simulink model "test"  (R2020b)
settings: Solver=ode4  StartTime=0.0  StopTime=inf  FixedStep=1/1000  RelTol=1e-3
libraries: speedgoatlib_IO691 x8, canmsglib x6, simulink x2
(part 1 of 2)
settings Model: SimulationMode=external  ExtModeEnableFloating=off  Creator=Mechatronics  LastModifiedBy=Mechatronics
settings SolverCC: ConcurrentTasks=on  PositivePriorityOrder=on
settings OptimizationCC: BlockReduction=off  OptimizeBlockIOStorage=off
settings DebuggingCC: TasksWithSamePriorityMsg=none
settings HardwareCC: ProdBitPerLong=64  ProdLongLongMode=on  ProdHWDeviceType=Intel->x86-64 (Linux 64)
settings RTWCC: Description=Simulink Real-Time  SystemTargetFile=slrealtime.tlc  TemplateMakefile=slrealtime_default_tmf  Toolchain=Simulink Real-Time Toolchain  BuildConfiguration=Faster Runs  CodeExecutionProfiling=on  TargetLang=C++

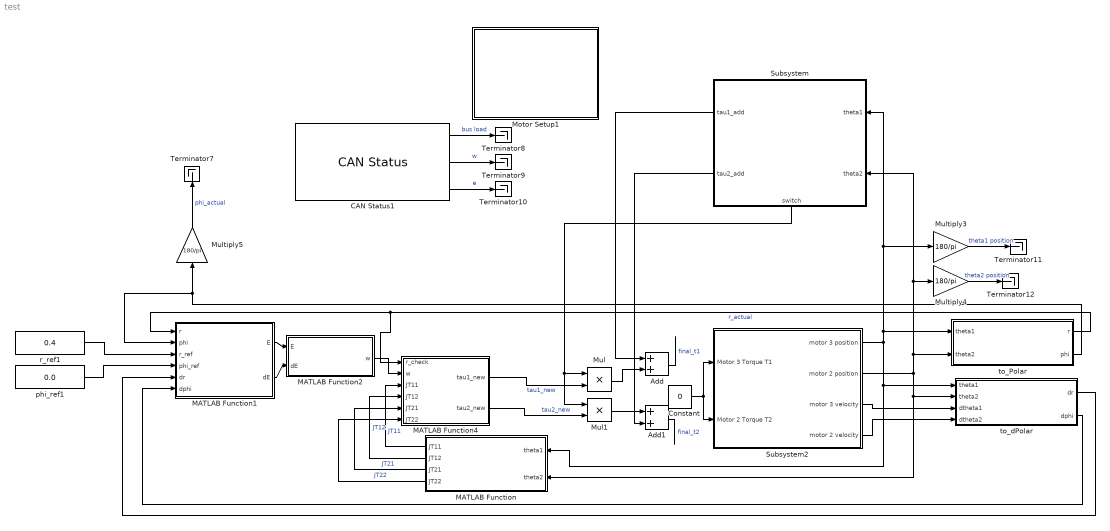
== system test ==
  Add : Sum
  Add1 : Sum
  CAN Status1 : speedgoatlib_IO691/CAN Status  moduleId=1  sampleTime=-1  channel=1  busRecovery=Off  arrayOutput=off  controllerCpuLoad=off  controllerLiveCount=off  initModeAct=off  avgBusLoad=on  receiving=off  RxQueueEmpty=off  dataOverrunRcv=off  rxBufferLevel=off  txPending=off  dataOverrunTx=off  txBufferLevel=off  errWarnLimit=on  errPassLimit=on  errBusOff=off  busRecoveryCounter=off  busCouplingErr=off  transceiverErr=off  opMode=off  brp=off  timeSegment1=off  timeSegment2=off  synchronisationJumpWidth=off  dataTSEG1=off  dataTSEG2=off  dataSJW=off  moduleType=691  qtyStatBlk=1  ptIdx=0  isFDMod=0
      settings: SourceProductName=Simulink Real-Time: Speedgoat I/O Blockset
  Constant : Constant  Value=0
  MATLAB Function : MATLAB Function  TreatAsAtomicUnit=on
  MATLAB Function1 : MATLAB Function  TreatAsAtomicUnit=on
  MATLAB Function2 : MATLAB Function  TreatAsAtomicUnit=on
  MATLAB Function4 : MATLAB Function  TreatAsAtomicUnit=on
  Motor Setup1 : Subsystem
  Mul : Product  Inputs=**
  Mul1 : Product  Inputs=**
  Multiply3 : Gain  Gain=180/pi
  Multiply4 : Gain  Gain=180/pi
  Multiply5 : Gain  Gain=180/pi
  Subsystem : Subsystem
      settings: PortSchema="{\"entries\":[{\"content\":{\"sides\":[{\"content\":{\"connectorIds\":[\"In1\",\"In2\"]},\"type\":\"ConnectorPlacement.EquallySpacedRectSide\",\"uuid\":\"133de2dd-f27a-4cc1-bddd-d1f84e4836c9\"},{\"content\":{\"connectorIds\":[\"Out1\",\"Out2\"],\"side\":\"RIGHT\"},\"type\":\"ConnectorPlacement.EquallySpacedRectSide\",\"uuid\":\"6569a8f1-8858-49fe-b592-3edc35f7d01c\"},{\"content\":{\"connectorIds\":[],\"side\":\"TOP\"},\"type\":\"ConnectorPlacement.EquallySpacedRectSide\",\"uuid\":\"dbb559e8-791c-4587-9e9a-4749d8cc79c6\"},{\"content\":{\"connectorIds\":[\"Out3\"],\"side\":\"BOTTOM\"},\"type\":\"ConnectorPlacement.EquallySpacedRectSide\",\"uuid\":\"b7c4d305-876d-4161-8903-ada4b7512b16\"},{\"content\":{\"connectorIds\":[],\"side\":\"HIDDEN\"},\"type\":\"ConnectorPlacement.EquallySpacedRectSide\",\"uuid\":\"a0aadd7d-61d3-4ce9-a370-27d87e201b6f\"}]},\"type\":\"ConnectorPlacement.EquallySpacedConnector\",\"uuid\":\"543a852a-1c67-4df2-af33-899992a7334e\"}],\"packageUris\":[\"http://schema.mathworks.com/mf0/Connector/R2020b\"],\"version\":\"1.0\"}"
  Subsystem2 : Subsystem
  Terminator{7..12} (6 alike) : Terminator
  phi_ref1 : Constant  Value=0.0
  r_ref1 : Constant  Value=0.4
  to_Polar : MATLAB Function  TreatAsAtomicUnit=on
  to_dPolar : MATLAB Function  TreatAsAtomicUnit=on
  wires:
  MATLAB Function4/2(tau2_new) -> Mul1/2  "tau2_new"
  Add/1 -> ?  "final_t1"
  Subsystem/3(switch) -> Mul1/1, Mul/1
  Multiply5/1 -> Terminator7/1  "phi_actual"
  Subsystem2/2(motor 2 position) -> to_dPolar/2(theta2), MATLAB Function/2(theta2), to_Polar/2(theta2), Subsystem/2(theta2), Multiply4/1
  MATLAB Function4/1(tau1_new) -> Mul/2  "tau1_new"
  Mul1/1 -> Add1/1
  MATLAB Function/4(JT22) -> MATLAB Function4/6(JT22)  "JT22"
  MATLAB Function/3(JT21) -> MATLAB Function4/5(JT21)  "JT21"
  MATLAB Function2/1(w) -> MATLAB Function4/2(w)
  Multiply4/1 -> Terminator12/1  "theta2 position"
  Multiply3/1 -> Terminator11/1  "theta1 position"
  MATLAB Function/2(JT12) -> MATLAB Function4/4(JT12)  "JT12"
  Subsystem/1(tau1_add) -> Add/1
  Subsystem2/3(motor 3 velocity) -> to_dPolar/3(dtheta1)
  Subsystem2/4(motor 2 velocity) -> to_dPolar/4(dtheta2)
  MATLAB Function/1(JT11) -> MATLAB Function4/3(JT11)  "JT11"
  Subsystem/2(tau2_add) -> Add1/2
  to_dPolar/1(dr) -> MATLAB Function1/5(dr)
  to_Polar/2(phi) -> MATLAB Function1/2(phi), Multiply5/1
  CAN Status1/1 -> Terminator8/1  "bus load"
  to_dPolar/2(dphi) -> MATLAB Function1/6(dphi)
  Subsystem2/1(motor 3 position) -> to_dPolar/1(theta1), MATLAB Function/1(theta1), to_Polar/1(theta1), Subsystem/1(theta1), Multiply3/1
  r_ref1/1 -> MATLAB Function1/3(r_ref)
  CAN Status1/3 -> Terminator10/1  "e"
  Add1/1 -> ?  "final_t2"
  MATLAB Function1/2(dE) -> MATLAB Function2/2(dE)
  MATLAB Function1/1(E) -> MATLAB Function2/1(E)
  to_Polar/1(r) -> MATLAB Function4/1(r_check), MATLAB Function1/1(r)  "r_actual"
  Mul/1 -> Add/2
  CAN Status1/2 -> Terminator9/1  "w"
  phi_ref1/1 -> MATLAB Function1/4(phi_ref)
  Constant/1 -> Subsystem2/2(Motor 2 Torque T2), Subsystem2/1(Motor 3 Torque T1)

== system test/Motor Setup1 ==
  CAN setup : speedgoatlib_IO691/CAN Setup   moduletype=IO691  id=1  pciSlot=-1  chn1=CAN (HS)  chn2=Disabled  chn3=Disabled  chn4=Disabled  initStruct=[]  termStruct=[struct('Channel',1,'Protocol','CAN','BRS',0,'Type','Standard','Identifier',2,'Data',[255, 255, 255, 255, 255, 255, 255, 253],'Pause',0.001), struct('Channel',1,'Protocol','CAN','BRS',0,'Type','Standard','Identifier',3,'Data',[255, 255, 255, 255, 255, 255, 255, 253],'Pause',0.001)]  ArbitrationbdrChn1=1.0 MBaud  ArbitrationManbdrChn1=[2,8,31,8]  FdbdrChn1=1.0 MBaud  FdManbdrChn1=[2,8,31,8]  ArbitrationbdrChn2=1.0 MBaud  ArbitrationManbdrChn2=[2,8,31,8]  FdbdrChn2=1.0 MBaud  FdManbdrChn2=[2,8,31,8]  ArbitrationbdrChn3=1.0 MBaud  ArbitrationManbdrChn3=[2,8,31,8]  FdbdrChn3=5.0 MBaud  FdManbdrChn3=[2,2,5,2]  ArbitrationbdrChn4=1.0 MBaud  ArbitrationManbdrChn4=[2,8,31,8]  FdbdrChn4=5.0 MBaud  FdManbdrChn4=[2,2,5,2]  moduleInitValues=[691 1 -1 -1]
      settings: SourceProductName=Simulink Real-Time: Speedgoat I/O Blockset
  Motor Setup : Subsystem

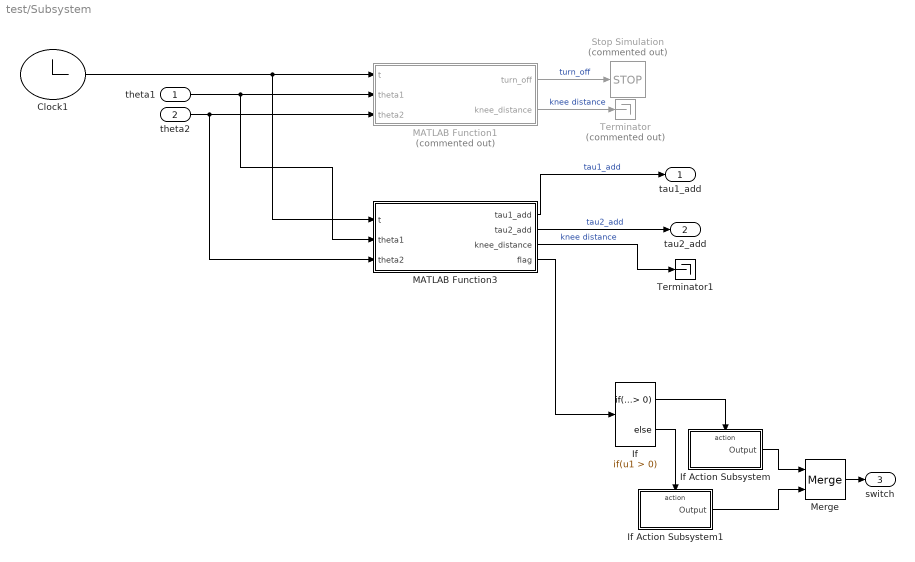
== system test/Subsystem ==
  theta1 : Inport
  theta2 : Inport  Port=2
  Clock1 : Clock
  If : If
  If Action Subsystem : Subsystem  TreatAsAtomicUnit=on
  If Action Subsystem1 : Subsystem  TreatAsAtomicUnit=on
  MATLAB Function1 : MATLAB Function  Commented=on  TreatAsAtomicUnit=on
  MATLAB Function3 : MATLAB Function  TreatAsAtomicUnit=on
  Merge : Merge
  Stop Simulation : Stop  Commented=on
  Terminator : Terminator  Commented=on
  Terminator1 : Terminator
  tau1_add : Outport
  tau2_add : Outport  Port=2
  switch : Outport  Port=3
  wires:
  theta2/1 -> MATLAB Function3/3(theta2), MATLAB Function1/3(theta2)
  theta1/1 -> MATLAB Function3/2(theta1), MATLAB Function1/2(theta1)
  MATLAB Function3/2(tau2_add) -> tau2_add/1  "tau2_add"
  MATLAB Function3/1(tau1_add) -> tau1_add/1  "tau1_add"
  MATLAB Function1/2(knee_distance) -> Terminator/1  "knee distance"
  MATLAB Function1/1(turn_off) -> Stop Simulation/1  "turn_off"
  Clock1/1 -> MATLAB Function3/1(t), MATLAB Function1/1(t)
  MATLAB Function3/3(knee_distance) -> Terminator1/1  "knee distance"
  If/2 -> If Action Subsystem1/Action
  If/1 -> If Action Subsystem/Action
  MATLAB Function3/4(flag) -> If/1
  If Action Subsystem/1(Output) -> Merge/1
  If Action Subsystem1/1(Output) -> Merge/2
  Merge/1 -> switch/1

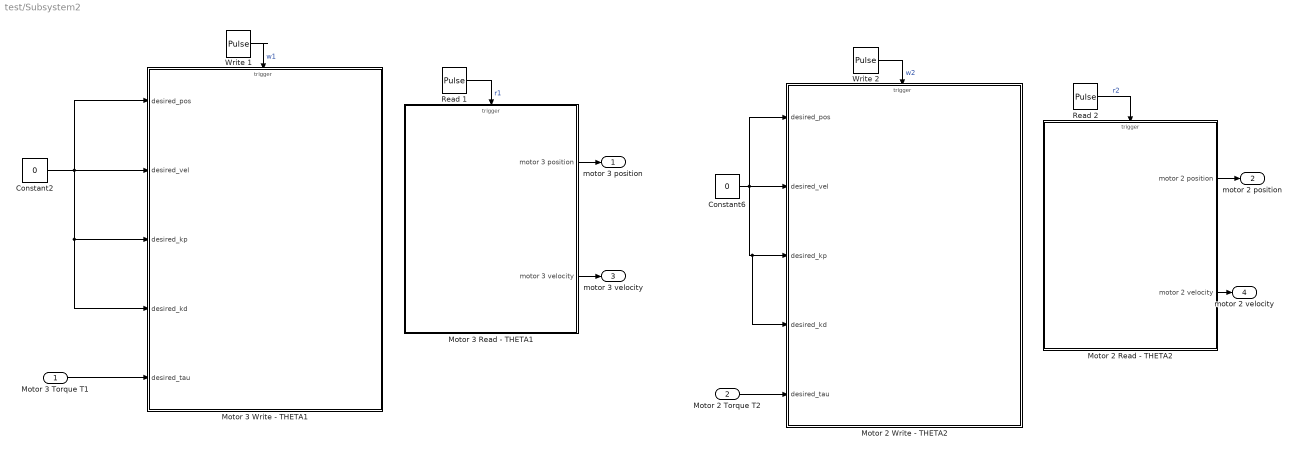
== system test/Subsystem2 ==
  Motor 3 Torque T1 : Inport
  Motor 2 Torque T2 : Inport  Port=2
  Constant2 : Constant  Value=0
  Constant6 : Constant  Value=0
  Motor 2 Read - THETA2 : Subsystem
  Motor 2 Write - THETA2 : Subsystem  TreatAsAtomicUnit=on
  Motor 3 Read - THETA1 : Subsystem
  Motor 3 Write - THETA1 : Subsystem  TreatAsAtomicUnit=on
  Read 1 : DiscretePulseGenerator  PulseType=Time based  Period=1/250  PulseWidth=50  PhaseDelay=3.001
  Read 2 : DiscretePulseGenerator  PulseType=Time based  Period=1/250  PulseWidth=50  PhaseDelay=3.003
  Write 1 : DiscretePulseGenerator  PulseType=Time based  Period=1/250  PulseWidth=50  PhaseDelay=3
  Write 2 : DiscretePulseGenerator  PulseType=Time based  Period=1/250  PulseWidth=50  PhaseDelay=3.002
  motor 3 position : Outport
  motor 2 position : Outport  Port=2
  motor 3 velocity : Outport  Port=3
  motor 2 velocity : Outport  Port=4
  wires:
  Motor 3 Read - THETA1/1(motor 3 position) -> motor 3 position/1
  Write 2/1 -> Motor 2 Write - THETA2/Trigger  "w2"
  Motor 2 Torque T2/1 -> Motor 2 Write - THETA2/5(desired_tau)
  Motor 2 Read - THETA2/2(motor 2 velocity) -> motor 2 velocity/1
  Motor 3 Read - THETA1/2(motor 3 velocity) -> motor 3 velocity/1
  Read 2/1 -> Motor 2 Read - THETA2/Trigger  "r2"
  Motor 3 Torque T1/1 -> Motor 3 Write - THETA1/5(desired_tau)
  Motor 2 Read - THETA2/1(motor 2 position) -> motor 2 position/1
  Read 1/1 -> Motor 3 Read - THETA1/Trigger  "r1"
  Write 1/1 -> Motor 3 Write - THETA1/Trigger  "w1"
  Constant6/1 -> Motor 2 Write - THETA2/1(desired_pos), Motor 2 Write - THETA2/4(desired_kd), Motor 2 Write - THETA2/3(desired_kp), Motor 2 Write - THETA2/2(desired_vel)
  Constant2/1 -> Motor 3 Write - THETA1/1(desired_pos), Motor 3 Write - THETA1/2(desired_vel), Motor 3 Write - THETA1/4(desired_kd), Motor 3 Write - THETA1/3(desired_kp)

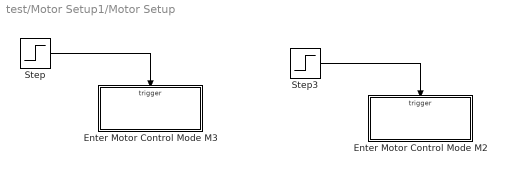
== system test/Motor Setup1/Motor Setup ==
  Enter Motor Control Mode M2 : Subsystem  TreatAsAtomicUnit=on
  Enter Motor Control Mode M3 : Subsystem  TreatAsAtomicUnit=on
  Step : Step  Time=1.0
  Step3 : Step  Time=2
  wires:
  Step3/1 -> Enter Motor Control Mode M2/Trigger
  Step/1 -> Enter Motor Control Mode M3/Trigger

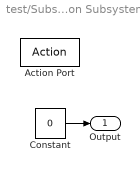
== system test/Subsystem/If Action Subsystem ==
  Action Port : ActionPort  ActionPortLabel=if(u1 > 0)
  Constant : Constant  Value=0
  Output : Outport
  wires:
  Constant/1 -> Output/1

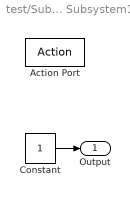
== system test/Subsystem/If Action Subsystem1 ==
  Action Port : ActionPort  ActionPortLabel=else
  Constant : Constant
  Output : Outport
  wires:
  Constant/1 -> Output/1

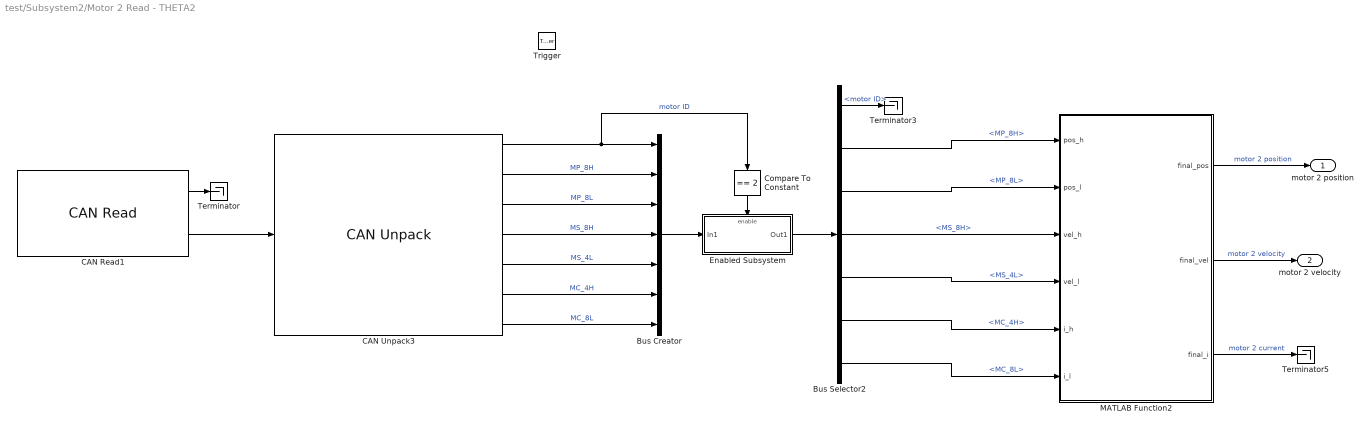
== system test/Subsystem2/Motor 2 Read - THETA2 ==
  Trigger : TriggerPort  VariantControl=Variant  PortDimensions=1
  Bus Creator : BusCreator  Inputs=7
  Bus Selector2 : BusSelector  OutputSignals=motor ID,MP_8H,MP_8L,MS_8H,MS_4L,MC_4H,MC_8L
  CAN Read1 : speedgoatlib_IO691/CAN Read  id=1  ts=-1  channel=1  messageType=CAN  canType=CAN (HS)  initValues=[691 1 -1 0 1 1]
      settings: SourceProductName=Simulink Real-Time: Speedgoat Library
  CAN Unpack3 : canmsglib/CAN Unpack  MsgList=(none)  MsgName=CAN Msg  MsgIDType=Standard (11-bit identifier)  MsgIdentifier=0  MsgLength=8  SignalInfo={ 'Drive ID', '0', '8', 'LE', 'unsigned', 'Standard', '0', '1', '0', '-Inf', 'Inf'; 'Motor position 8-H', '8', '8', 'LE', 'unsigned', 'Standard', '0', '1', '0', '-Inf', 'Inf'; 'Motor position 8-L', '16', '8', 'LE', 'unsigned', 'Standard', '0', '1', '0', '-Inf', 'Inf'; 'Motor speed 8-H', '24', '8', 'LE', 'unsigned', 'Standard', '0', '1', '0', '-Inf', 'Inf'; 'Motor speed 4-L', '36', '4', 'LE', 'unsigned', 'Standard', '0', '1', '0', '-Inf', 'Inf'; 'Current 4-H', '32', '4', 'LE', 'unsigned', 'Standard', '0', '1', '0', '-Inf', 'Inf'; 'Current 8-L', '40', '8', 'LE', 'unsigned', 'Standard', '0', '1', '0', '-Inf', 'Inf' }  IDPort=off  TimestampPort=off  ErrorPort=off  RemotePort=off  LengthPort=off  StatusPort=off  ApplyMinMax=off
      settings: SourceProductBaseCode=ME,XP,VN
  Compare To Constant : simulink/Logic and Bit Operations/Compare To Constant  relop===  const=2  OutDataTypeStr=boolean
  Enabled Subsystem : Subsystem  TreatAsAtomicUnit=on
  MATLAB Function2 : MATLAB Function  TreatAsAtomicUnit=on
  Terminator : Terminator
  Terminator3 : Terminator
  Terminator5 : Terminator
  motor 2 position : Outport
  motor 2 velocity : Outport  Port=2
  wires:
  MATLAB Function2/3(final_i) -> Terminator5/1  "motor 2 current"
  MATLAB Function2/1(final_pos) -> motor 2 position/1  "motor 2 position"
  MATLAB Function2/2(final_vel) -> motor 2 velocity/1  "motor 2 velocity"
  CAN Unpack3/7 -> Bus Creator/7  "MC_8L"
  Bus Selector2/4 -> MATLAB Function2/3(vel_h)  "<MS_8H>"
  Bus Selector2/7 -> MATLAB Function2/6(i_l)  "<MC_8L>"
  CAN Unpack3/4 -> Bus Creator/4  "MS_8H"
  CAN Unpack3/6 -> Bus Creator/6  "MC_4H"
  Bus Selector2/1 -> Terminator3/1  "<motor ID>"
  CAN Unpack3/3 -> Bus Creator/3  "MP_8L"
  Bus Selector2/2 -> MATLAB Function2/1(pos_h)  "<MP_8H>"
  Bus Selector2/5 -> MATLAB Function2/4(vel_l)  "<MS_4L>"
  CAN Unpack3/2 -> Bus Creator/2  "MP_8H"
  CAN Read1/2 -> CAN Unpack3/1
  CAN Unpack3/5 -> Bus Creator/5  "MS_4L"
  Bus Selector2/6 -> MATLAB Function2/5(i_h)  "<MC_4H>"
  Bus Selector2/3 -> MATLAB Function2/2(pos_l)  "<MP_8L>"
  Compare To Constant/1 -> Enabled Subsystem/Enable
  Bus Creator/1 -> Enabled Subsystem/1(In1)
  CAN Unpack3/1 -> Compare To Constant/1, Bus Creator/1  "motor ID"
  Enabled Subsystem/1(Out1) -> Bus Selector2/1
  CAN Read1/1 -> Terminator/1

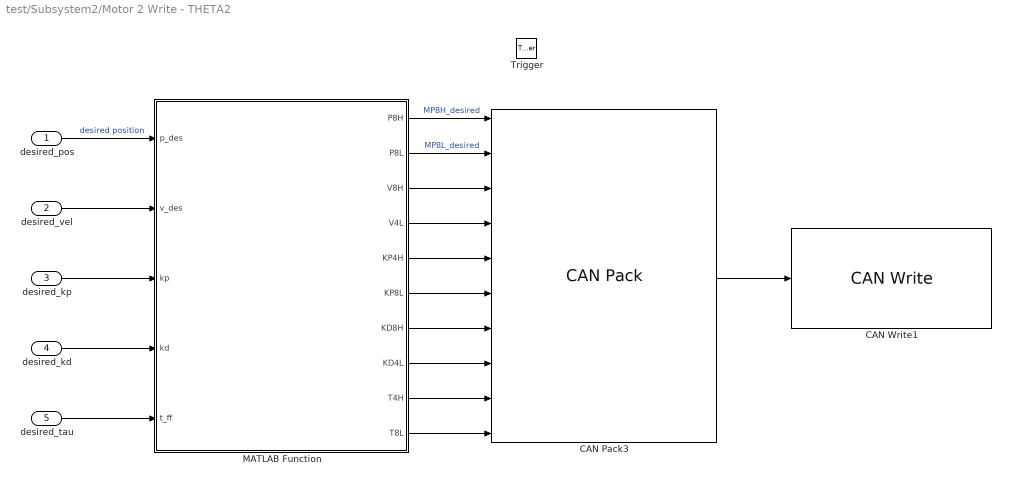
== system test/Subsystem2/Motor 2 Write - THETA2 ==
  desired_pos : Inport
  desired_vel : Inport  Port=2
  desired_kp : Inport  Port=3
  desired_kd : Inport  Port=4
  desired_tau : Inport  Port=5
  Trigger : TriggerPort  VariantControl=Variant
  CAN Pack3 : canmsglib/CAN Pack  MsgList=(none)  MsgName=MotorControl  MsgIDType=Standard (11-bit identifier)  MsgIdentifier=2  MsgLength=8  Remote=off  ApplyMinMax=off  BusOutput=off  SignalInfo={ 'Motor postition 8-H', '0', '8', 'LE', 'unsigned', 'Standard', '0', '1', '0', '-Inf', 'Inf'; 'Motor position 8-L', '8', '8', 'LE', 'unsigned', 'Standard', '0', '1', '0', '-Inf', 'Inf'; 'Motor speed 8-H', '16', '8', 'LE', 'unsigned', 'Standard', '0', '1', '0', '-Inf', 'Inf'; 'Motor speed 4-L', '28', '4', 'LE', 'unsigned', 'Standard', '0', '1', '0', '-Inf', 'Inf'; 'KP 4-H', '24', '4', 'LE', 'unsigned', 'Standard', '0', '1', '0', '-Inf', 'Inf'; 'KP 8-L', '32', '8', 'LE', 'unsigned', 'Standard', '0', '1', '0', '-Inf', 'Inf'; 'KD 8-H', '40', '8', 'LE', 'unsigned', 'Standard', '0', '1', '0', '-Inf', 'Inf'; 'KD 4-L', '52', '4', 'LE', 'unsigned', 'Standard', '0', '1', '0', '-Inf', 'Inf'; 'Current 4-H', '48', '4', 'LE', 'unsigned', 'Standard', '0', '1', '0', '-Inf', 'Inf'; 'Current 8-L', '56', '8', 'LE', 'unsigned', 'Standard', '0', '1', '0', '-Inf', 'Inf' }
      settings: SourceProductBaseCode=ME,XP,VN  DataFormat=manually specified signals
  CAN Write1 : speedgoatlib_IO691/CAN Write  id=1  ts=-1  channel=1  messageType=CAN  enableStatusPort=off  canType=CAN (HS)  initValues=[691 1 -1 0 1 1 0]
      settings: SourceProductName=Simulink Real-Time: Speedgoat Library
  MATLAB Function : MATLAB Function  TreatAsAtomicUnit=on
  wires:
  desired_vel/1 -> MATLAB Function/2(v_des)
  desired_pos/1 -> MATLAB Function/1(p_des)  "desired position"
  MATLAB Function/6(KP8L) -> CAN Pack3/6
  MATLAB Function/7(KD8H) -> CAN Pack3/7
  MATLAB Function/2(P8L) -> CAN Pack3/2  "MP8L_desired"
  desired_kp/1 -> MATLAB Function/3(kp)
  MATLAB Function/5(KP4H) -> CAN Pack3/5
  desired_kd/1 -> MATLAB Function/4(kd)
  desired_tau/1 -> MATLAB Function/5(t_ff)
  MATLAB Function/8(KD4L) -> CAN Pack3/8
  MATLAB Function/4(V4L) -> CAN Pack3/4
  MATLAB Function/9(T4H) -> CAN Pack3/9
  MATLAB Function/1(P8H) -> CAN Pack3/1  "MP8H_desired"
  CAN Pack3/1 -> CAN Write1/1
  MATLAB Function/3(V8H) -> CAN Pack3/3
  MATLAB Function/10(T8L) -> CAN Pack3/10

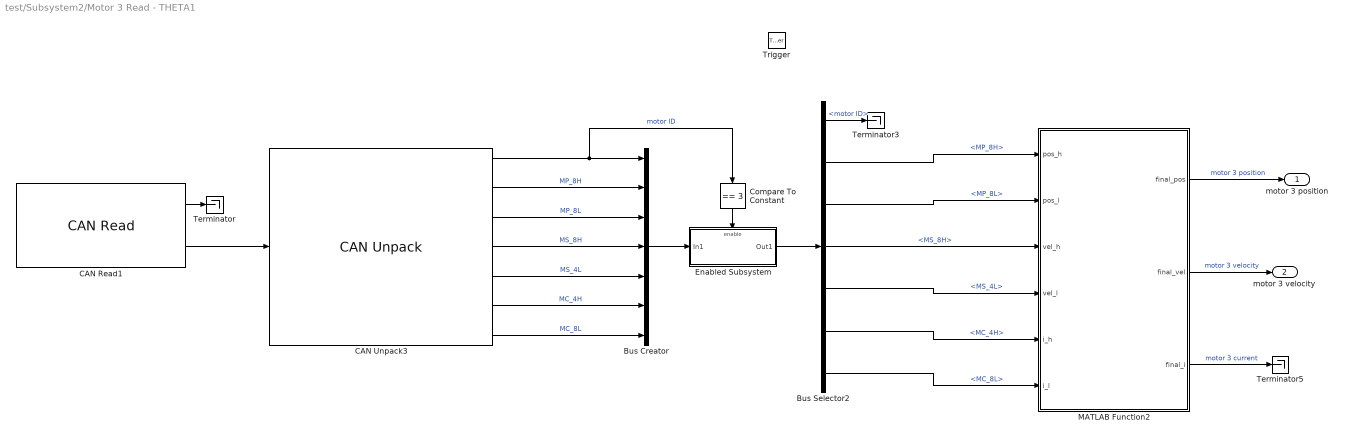
== system test/Subsystem2/Motor 3 Read - THETA1 ==
  Trigger : TriggerPort  VariantControl=Variant  PortDimensions=1
  Bus Creator : BusCreator  Inputs=7
  Bus Selector2 : BusSelector  OutputSignals=motor ID,MP_8H,MP_8L,MS_8H,MS_4L,MC_4H,MC_8L
  CAN Read1 : speedgoatlib_IO691/CAN Read  id=1  ts=-1  channel=1  messageType=CAN  canType=CAN (HS)  initValues=[691 1 -1 0 1 1]
      settings: SourceProductName=Simulink Real-Time: Speedgoat Library
  CAN Unpack3 : canmsglib/CAN Unpack  MsgList=(none)  MsgName=CAN Msg  MsgIDType=Standard (11-bit identifier)  MsgIdentifier=0  MsgLength=8  SignalInfo={ 'Drive ID', '0', '8', 'LE', 'unsigned', 'Standard', '0', '1', '0', '-Inf', 'Inf'; 'Motor position 8-H', '8', '8', 'LE', 'unsigned', 'Standard', '0', '1', '0', '-Inf', 'Inf'; 'Motor position 8-L', '16', '8', 'LE', 'unsigned', 'Standard', '0', '1', '0', '-Inf', 'Inf'; 'Motor speed 8-H', '24', '8', 'LE', 'unsigned', 'Standard', '0', '1', '0', '-Inf', 'Inf'; 'Motor speed 4-L', '36', '4', 'LE', 'unsigned', 'Standard', '0', '1', '0', '-Inf', 'Inf'; 'Current 4-H', '32', '4', 'LE', 'unsigned', 'Standard', '0', '1', '0', '-Inf', 'Inf'; 'Current 8-L', '40', '8', 'LE', 'unsigned', 'Standard', '0', '1', '0', '-Inf', 'Inf' }  IDPort=off  TimestampPort=off  ErrorPort=off  RemotePort=off  LengthPort=off  StatusPort=off  ApplyMinMax=off
      settings: SourceProductBaseCode=ME,XP,VN
  Compare To Constant : simulink/Logic and Bit Operations/Compare To Constant  relop===  const=3  OutDataTypeStr=boolean
  Enabled Subsystem : Subsystem  TreatAsAtomicUnit=on
  MATLAB Function2 : MATLAB Function  TreatAsAtomicUnit=on
  Terminator : Terminator
  Terminator3 : Terminator
  Terminator5 : Terminator
  motor 3 position : Outport
  motor 3 velocity : Outport  Port=2
  wires:
  MATLAB Function2/3(final_i) -> Terminator5/1  "motor 3 current"
  MATLAB Function2/1(final_pos) -> motor 3 position/1  "motor 3 position"
  MATLAB Function2/2(final_vel) -> motor 3 velocity/1  "motor 3 velocity"
  CAN Unpack3/7 -> Bus Creator/7  "MC_8L"
  Bus Selector2/4 -> MATLAB Function2/3(vel_h)  "<MS_8H>"
  Bus Selector2/7 -> MATLAB Function2/6(i_l)  "<MC_8L>"
  CAN Unpack3/4 -> Bus Creator/4  "MS_8H"
  CAN Unpack3/6 -> Bus Creator/6  "MC_4H"
  Bus Selector2/1 -> Terminator3/1  "<motor ID>"
  CAN Unpack3/3 -> Bus Creator/3  "MP_8L"
  Bus Selector2/2 -> MATLAB Function2/1(pos_h)  "<MP_8H>"
  Bus Selector2/5 -> MATLAB Function2/4(vel_l)  "<MS_4L>"
  CAN Unpack3/2 -> Bus Creator/2  "MP_8H"
  CAN Read1/2 -> CAN Unpack3/1
  CAN Unpack3/5 -> Bus Creator/5  "MS_4L"
  Bus Selector2/6 -> MATLAB Function2/5(i_h)  "<MC_4H>"
  Bus Selector2/3 -> MATLAB Function2/2(pos_l)  "<MP_8L>"
  Compare To Constant/1 -> Enabled Subsystem/Enable
  Bus Creator/1 -> Enabled Subsystem/1(In1)
  CAN Unpack3/1 -> Compare To Constant/1, Bus Creator/1  "motor ID"
  Enabled Subsystem/1(Out1) -> Bus Selector2/1
  CAN Read1/1 -> Terminator/1

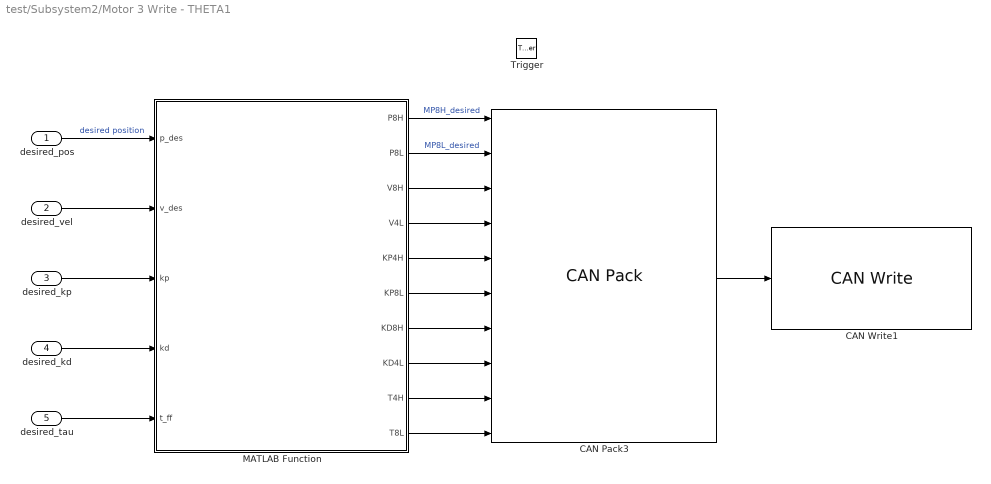
== system test/Subsystem2/Motor 3 Write - THETA1 ==
  desired_pos : Inport
  desired_vel : Inport  Port=2
  desired_kp : Inport  Port=3
  desired_kd : Inport  Port=4
  desired_tau : Inport  Port=5
  Trigger : TriggerPort  VariantControl=Variant
  CAN Pack3 : canmsglib/CAN Pack  MsgList=(none)  MsgName=MotorControl  MsgIDType=Standard (11-bit identifier)  MsgIdentifier=3  MsgLength=8  Remote=off  ApplyMinMax=off  BusOutput=off  SignalInfo={ 'Motor postition 8-H', '0', '8', 'LE', 'unsigned', 'Standard', '0', '1', '0', '-Inf', 'Inf'; 'Motor position 8-L', '8', '8', 'LE', 'unsigned', 'Standard', '0', '1', '0', '-Inf', 'Inf'; 'Motor speed 8-H', '16', '8', 'LE', 'unsigned', 'Standard', '0', '1', '0', '-Inf', 'Inf'; 'Motor speed 4-L', '28', '4', 'LE', 'unsigned', 'Standard', '0', '1', '0', '-Inf', 'Inf'; 'KP 4-H', '24', '4', 'LE', 'unsigned', 'Standard', '0', '1', '0', '-Inf', 'Inf'; 'KP 8-L', '32', '8', 'LE', 'unsigned', 'Standard', '0', '1', '0', '-Inf', 'Inf'; 'KD 8-H', '40', '8', 'LE', 'unsigned', 'Standard', '0', '1', '0', '-Inf', 'Inf'; 'KD 4-L', '52', '4', 'LE', 'unsigned', 'Standard', '0', '1', '0', '-Inf', 'Inf'; 'Current 4-H', '48', '4', 'LE', 'unsigned', 'Standard', '0', '1', '0', '-Inf', 'Inf'; 'Current 8-L', '56', '8', 'LE', 'unsigned', 'Standard', '0', '1', '0', '-Inf', 'Inf' }
      settings: SourceProductBaseCode=ME,XP,VN  DataFormat=manually specified signals
  CAN Write1 : speedgoatlib_IO691/CAN Write  id=1  ts=-1  channel=1  messageType=CAN  enableStatusPort=off  canType=CAN (HS)  initValues=[691 1 -1 0 1 1 0]
      settings: SourceProductName=Simulink Real-Time: Speedgoat I/O Blockset
  MATLAB Function : MATLAB Function  TreatAsAtomicUnit=on
  wires:
  desired_vel/1 -> MATLAB Function/2(v_des)
  desired_pos/1 -> MATLAB Function/1(p_des)  "desired position"
  MATLAB Function/6(KP8L) -> CAN Pack3/6
  MATLAB Function/7(KD8H) -> CAN Pack3/7
  MATLAB Function/2(P8L) -> CAN Pack3/2  "MP8L_desired"
  desired_kp/1 -> MATLAB Function/3(kp)
  MATLAB Function/5(KP4H) -> CAN Pack3/5
  desired_kd/1 -> MATLAB Function/4(kd)
  desired_tau/1 -> MATLAB Function/5(t_ff)
  MATLAB Function/8(KD4L) -> CAN Pack3/8
  MATLAB Function/4(V4L) -> CAN Pack3/4
  MATLAB Function/9(T4H) -> CAN Pack3/9
  MATLAB Function/1(P8H) -> CAN Pack3/1  "MP8H_desired"
  CAN Pack3/1 -> CAN Write1/1
  MATLAB Function/3(V8H) -> CAN Pack3/3
  MATLAB Function/10(T8L) -> CAN Pack3/10

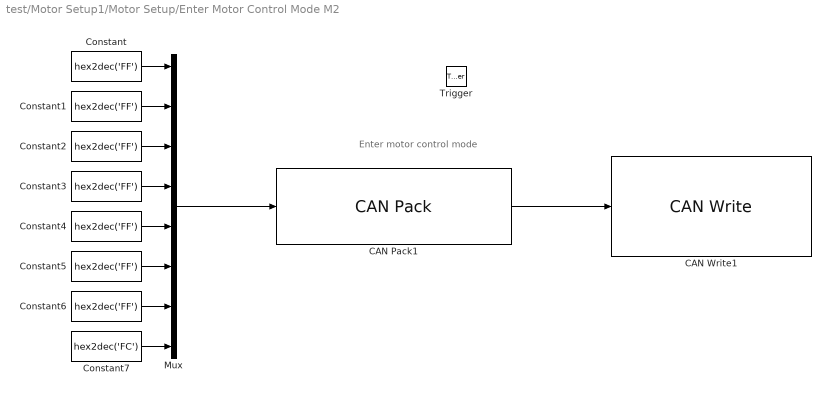
== system test/Motor Setup1/Motor Setup/Enter Motor Control Mode M2 ==
  note: Enter motor control mode
  Trigger : TriggerPort  VariantControl=Variant
  CAN Pack1 : canmsglib/CAN Pack  MsgList=(none)  MsgName=CAN Msg  MsgIDType=Standard (11-bit identifier)  MsgIdentifier=2  MsgLength=8  Remote=off  ApplyMinMax=off  BusOutput=off  SignalInfo={ 'Motor postition 8-H', '0', '8', 'LE', 'unsigned', 'Standard', '0', '1', '0', '-Inf', 'Inf'; 'Motor position 8-L', '8', '8', 'LE', 'unsigned', 'Standard', '0', '1', '0', '-Inf', 'Inf'; 'Motor seed 8-H', '16', '8', 'LE', 'unsigned', 'Standard', '0', '1', '0', '-Inf', 'Inf'; 'Motor speed 4-L', '28', '4', 'LE', 'unsigned', 'Standard', '0', '1', '0', '-Inf', 'Inf'; 'KP 4-H', '24', '4', 'LE', 'unsigned', 'Standard', '0', '1', '0', '-Inf', 'Inf'; 'KP 8-L', '32', '8', 'LE', 'unsigned', 'Standard', '0', '1', '0', '-Inf', 'Inf'; 'KP 8-H', '40', '8', 'LE', 'unsigned', 'Standard', '0', '1', '0', '-Inf', 'Inf'; 'KD 4-L', '52', '4', 'LE', 'unsigned', 'Standard', '0', '1', '0', '-Inf', 'Inf'; 'Current 4-H', '48', '4', 'LE', 'unsigned', 'Standard', '0', '1', '0', '-Inf', 'Inf'; 'Current 8-L', '56', '8', 'LE', 'unsigned', 'Standard', '0', '1', '0', '-Inf', 'Inf' }
      settings: SourceProductBaseCode=ME,XP,VN  DataFormat=raw data
  CAN Write1 : speedgoatlib_IO691/CAN Write  id=1  ts=-1  channel=1  messageType=CAN  enableStatusPort=off  canType=CAN (HS)  initValues=[691 1 -1 0 1 1 0]
      settings: SourceProductName=Simulink Real-Time: Speedgoat Library
  Constant{,1..6} (7 alike) : Constant  Value=hex2dec('FF')  OutDataTypeStr=uint8  SampleTime=-1
  Constant7 : Constant  Value=hex2dec('FC')  OutDataTypeStr=uint8  SampleTime=-1
  Mux : Mux  Inputs=8
  wires:
  CAN Pack1/1 -> CAN Write1/1
  Mux/1 -> CAN Pack1/1
  Constant7/1 -> Mux/8
  Constant4/1 -> Mux/5
  Constant1/1 -> Mux/2
  Constant5/1 -> Mux/6
  Constant3/1 -> Mux/4
  Constant2/1 -> Mux/3
  Constant/1 -> Mux/1
  Constant6/1 -> Mux/7

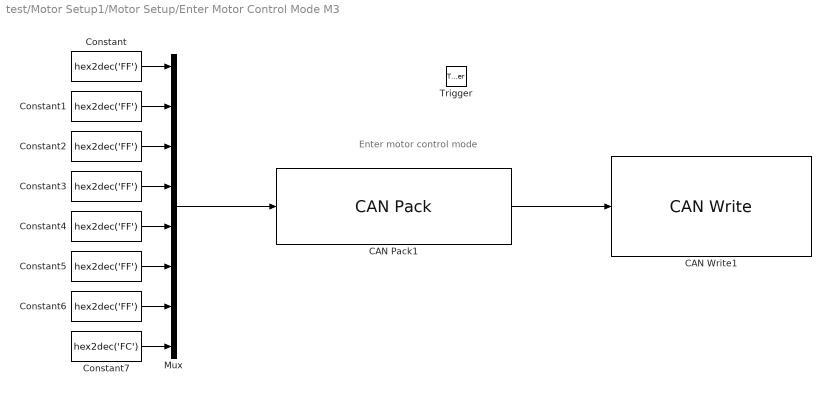
== system test/Motor Setup1/Motor Setup/Enter Motor Control Mode M3 ==
  note: Enter motor control mode
  Trigger : TriggerPort  VariantControl=Variant
  CAN Pack1 : canmsglib/CAN Pack  MsgList=(none)  MsgName=CAN Msg  MsgIDType=Standard (11-bit identifier)  MsgIdentifier=3  MsgLength=8  Remote=off  ApplyMinMax=off  BusOutput=off  SignalInfo={ 'Motor postition 8-H', '0', '8', 'LE', 'unsigned', 'Standard', '0', '1', '0', '-Inf', 'Inf'; 'Motor position 8-L', '8', '8', 'LE', 'unsigned', 'Standard', '0', '1', '0', '-Inf', 'Inf'; 'Motor seed 8-H', '16', '8', 'LE', 'unsigned', 'Standard', '0', '1', '0', '-Inf', 'Inf'; 'Motor speed 4-L', '28', '4', 'LE', 'unsigned', 'Standard', '0', '1', '0', '-Inf', 'Inf'; 'KP 4-H', '24', '4', 'LE', 'unsigned', 'Standard', '0', '1', '0', '-Inf', 'Inf'; 'KP 8-L', '32', '8', 'LE', 'unsigned', 'Standard', '0', '1', '0', '-Inf', 'Inf'; 'KP 8-H', '40', '8', 'LE', 'unsigned', 'Standard', '0', '1', '0', '-Inf', 'Inf'; 'KD 4-L', '52', '4', 'LE', 'unsigned', 'Standard', '0', '1', '0', '-Inf', 'Inf'; 'Current 4-H', '48', '4', 'LE', 'unsigned', 'Standard', '0', '1', '0', '-Inf', 'Inf'; 'Current 8-L', '56', '8', 'LE', 'unsigned', 'Standard', '0', '1', '0', '-Inf', 'Inf' }
      settings: SourceProductBaseCode=ME,XP,VN  DataFormat=raw data
  CAN Write1 : speedgoatlib_IO691/CAN Write  id=1  ts=-1  channel=1  messageType=CAN  enableStatusPort=off  canType=CAN (HS)  initValues=[691 1 -1 0 1 1 0]
      settings: SourceProductName=Simulink Real-Time: Speedgoat Library
  Constant{,1..6} (7 alike) : Constant  Value=hex2dec('FF')  OutDataTypeStr=uint8  SampleTime=-1
  Constant7 : Constant  Value=hex2dec('FC')  OutDataTypeStr=uint8  SampleTime=-1
  Mux : Mux  Inputs=8
  wires:
  CAN Pack1/1 -> CAN Write1/1
  Mux/1 -> CAN Pack1/1
  Constant7/1 -> Mux/8
  Constant4/1 -> Mux/5
  Constant1/1 -> Mux/2
  Constant5/1 -> Mux/6
  Constant3/1 -> Mux/4
  Constant2/1 -> Mux/3
  Constant/1 -> Mux/1
  Constant6/1 -> Mux/7

== system test/Subsystem2/Motor 2 Read - THETA2/Enabled Subsystem ==
  In1 : Inport
  Enable : EnablePort
  Out1 : Outport
  wires:
  In1/1 -> Out1/1

== system test/Subsystem2/Motor 3 Read - THETA1/Enabled Subsystem ==
  In1 : Inport
  Enable : EnablePort
  Out1 : Outport
  wires:
  In1/1 -> Out1/1

== matlab function test/Subsystem2/Motor 3 Write - THETA1/MATLAB Function ==
  data: p_des input; P8H output; v_des input; kp input; kd input; t_ff input; P8L output; V8H output; V4L output; KP4H output; KP8L output; KD8H output; KD4L output; T4H output; T8L output
function [P8H,P8L,V8H,V4L,KP4H,KP8L,KD8H,KD4L,T4H,T8L] = AK1090(p_des, v_des, kp, kd, t_ff)
    % Coppied from AK70-10 manual
    % NB: CONSTANTS FOR AK70-10
    p_min = -12.5; % rad
    p_max = +12.5; % rad
    v_min = -50.0; % rad/s
    v_max = +50.0; % rad/s
    t_min = -65.0; % Nm
    t_max = +65.0; % Nm
    kp_min = 0;
    kp_max = 500;
    kd_min = 0;
    kd_max = 5;
    
    % bound inputs
    p_des = min([max([p_min,p_des]),p_max]);
    v_des = min([max([v_min,v_des]),v_max]);
    kp = min([max([kp_min,kp]),kp_max]);
    kd = min([max([kd_min,kd]),kd_max]);
    t_ff = min([max([t_min,t_ff]),t_max]);
    
    % convert floats to unsigned integers
    p_int = float_to_uint(p_des, p_min, p_max, 16);
    v_int = float_to_uint(v_des, v_min, v_max, 12);
    kp_int = float_to_uint(kp, kp_min, kp_max, 12);
    kd_int = float_to_uint(kd, kd_min, kd_max, 12);
    t_int = float_to_uint(t_ff, t_min, t_max, 12);
    
    % break up for CAN frame 
    P8H = bitshift(p_int, -8); % 8 higher bits
    P8L = bitand(p_int, 0xFF); % 8 lower bits
    V8H = bitshift(v_int, -4); % 8 higher bits
    V4L = bitand(v_int, 0xF); % 4 lower bits
    KP4H = bitshift(kp_int, -8); % 4 higher bits
    KP8L = bitand(kp_int, 0xFF); % 8 lower bits
    KD8H = bitshift(kd_int, -4); % 8 higher bits
    KD4L = bitand(kd_int, 0xF); % 4 lower bits
    T4H = bitshift(t_int, -8); % 4 higher bits
    T8L = bitand(t_int, 0xFF); % 8 lower bits
    
    % Converts a float to an unsigned int, given range and number of bits
    function x_int = float_to_uint(x, x_min, x_max, n_bits)
        span = x_max - x_min;
        min([max([x_min,x]),x_max])
        x_int = ((x - x_min)*(bitshift(1, n_bits) / span));
    end
end
%final_values = desired_pos,desired_vel,desired_kp,desired_kd,desired_tau;

== matlab function test/Subsystem2/Motor 2 Write - THETA2/MATLAB Function ==
  data: p_des input; P8H output; v_des input; kp input; kd input; t_ff input; P8L output; V8H output; V4L output; KP4H output; KP8L output; KD8H output; KD4L output; T4H output; T8L output
function [P8H,P8L,V8H,V4L,KP4H,KP8L,KD8H,KD4L,T4H,T8L] = AK1090(p_des, v_des, kp, kd, t_ff)
    % Coppied from AK70-10 manual
    % NB: CONSTANTS FOR AK70-10
    p_min = -12.5; % rad
    p_max = +12.5; % rad
    v_min = -50.0; % rad/s
    v_max = +50.0; % rad/s
    t_min = -65.0; % Nm
    t_max = +65.0; % Nm
    kp_min = 0;
    kp_max = 500;
    kd_min = 0;
    kd_max = 5;
    
    % bound inputs
    p_des = min([max([p_min,p_des]),p_max]);
    v_des = min([max([v_min,v_des]),v_max]);
    kp = min([max([kp_min,kp]),kp_max]);
    kd = min([max([kd_min,kd]),kd_max]);
    t_ff = min([max([t_min,t_ff]),t_max]);
    
    % convert floats to unsigned integers
    p_int = float_to_uint(p_des, p_min, p_max, 16);
    v_int = float_to_uint(v_des, v_min, v_max, 12);
    kp_int = float_to_uint(kp, kp_min, kp_max, 12);
    kd_int = float_to_uint(kd, kd_min, kd_max, 12);
    t_int = float_to_uint(t_ff, t_min, t_max, 12);
    
    % break up for CAN frame 
    P8H = bitshift(p_int, -8); % 8 higher bits
    P8L = bitand(p_int, 0xFF); % 8 lower bits
    V8H = bitshift(v_int, -4); % 8 higher bits
    V4L = bitand(v_int, 0xF); % 4 lower bits
    KP4H = bitshift(kp_int, -8); % 4 higher bits
    KP8L = bitand(kp_int, 0xFF); % 8 lower bits
    KD8H = bitshift(kd_int, -4); % 8 higher bits
    KD4L = bitand(kd_int, 0xF); % 4 lower bits
    T4H = bitshift(t_int, -8); % 4 higher bits
    T8L = bitand(t_int, 0xFF); % 8 lower bits
    
    % Converts a float to an unsigned int, given range and number of bits
    function x_int = float_to_uint(x, x_min, x_max, n_bits)
        span = x_max - x_min;
        min([max([x_min,x]),x_max])
        x_int = ((x - x_min)*(bitshift(1, n_bits) / span));
    end
end
%final_values = desired_pos,desired_vel,desired_kp,desired_kd,desired_tau;

== matlab function test/Subsystem2/Motor 2 Read - THETA2/MATLAB Function2 ==
  data: pos_h input; final_pos output; pos_l input; vel_h input; vel_l input; i_h input; i_l input; final_vel output; final_i output
function [final_pos,final_vel,final_i] = fcn(pos_h,pos_l,vel_h,vel_l,i_h,i_l)
% ------------------------------------
max_pos = 12.5;
min_pos = -12.5;
span_pos = max_pos - min_pos;
offset_pos = max_pos;

pos = bitshift(pos_h,8);
combined_pos = bitor(pos,pos_l);

range_pos = ((combined_pos*span_pos)/(2^16-1))-offset_pos;

final_pos = (range_pos*4*pi)/12.5;
% ------------------------------------
max_vel = 23.24;
min_vel = -23.24;
span_vel = max_vel - min_vel;
offset_vel = max_vel;
vel = bitshift(vel_h,4);
combined_vel = bitor(vel,vel_l);

final_vel = ((combined_vel*span_vel)/(2^12-1))-offset_vel;

% ------------------------------------
max_i = 54;
min_i = -54;
span_i = max_i - min_i;
offset_i = max_i;
i = bitshift(i_h,8);
combined_i = bitor(i,i_l);

final_i = ((combined_i*span_i)/(2^12-1))-offset_i;
end

== matlab function test/Subsystem2/Motor 3 Read - THETA1/MATLAB Function2 ==
  data: pos_h input; final_pos output; pos_l input; vel_h input; vel_l input; i_h input; i_l input; final_vel output; final_i output
function [final_pos,final_vel,final_i] = fcn(pos_h,pos_l,vel_h,vel_l,i_h,i_l)
% ------------------------------------
max_pos = 12.5;
min_pos = -12.5;
span_pos = max_pos - min_pos;
offset_pos = max_pos;

pos = bitshift(pos_h,8);
combined_pos = bitor(pos,pos_l);

range_pos = ((combined_pos*span_pos)/(2^16-1))-offset_pos;

final_pos = (range_pos*4*pi)/12.5;
% ------------------------------------
max_vel = 23.24;
min_vel = -23.24;
span_vel = max_vel - min_vel;
offset_vel = max_vel;
vel = bitshift(vel_h,4);
combined_vel = bitor(vel,vel_l);

final_vel = ((combined_vel*span_vel)/(2^12-1))-offset_vel;

% ------------------------------------
max_i = 54;
min_i = -54;
span_i = max_i - min_i;
offset_i = max_i;
i = bitshift(i_h,8);
combined_i = bitor(i,i_l);

final_i = ((combined_i*span_i)/(2^12-1))-offset_i;
end

== matlab function test/Subsystem/MATLAB Function3 ==
  data: t input; theta1 input; tau1_add output; theta2 input; tau2_add output; knee_distance output; flag output
function [tau1_add,tau2_add,knee_distance,flag] = PUSH(t,theta1,theta2)
    % End simulation if knees are too close 
    L1 = 18.5/100;
    L2 = 18.5/100;
    L5 = 12/100;
    q1 =  pi/2 - theta1; 
    q2 =  pi/2 - theta2;
    B1 = [-0.5*L5 - L1*cos(q1) ; L1*sin(q1)];
    B2 = [0.5*L5 + L2*cos(pi-q2) ; L2*sin(pi-q2)];
    knee_distance = abs(B1(1) - B2(1));
    if knee_distance<=0.12
        if t>=3.5
            tau1_add = 3;
            tau2_add = -3;
            flag = 1;
        else 
            tau1_add = 0;
            tau2_add = 0;
            flag = 0;
        end
    else 
        tau1_add = 0;
        tau2_add = 0;
        flag = 0;
    end

end

== matlab function test/MATLAB Function1 ==
  data: E output; r input; phi input; r_ref input; phi_ref input; dE output; dr input; dphi input
function [E,dE] = Error(r,phi,r_ref,phi_ref,dr,dphi)
    
    dr_ref = 0.0;
    dphi_ref = 0.0;
    
    E = [r_ref - r; phi_ref - phi];
    dE = [dr_ref - dr; dphi_ref - dphi];
    
end

== matlab function test/to_Polar ==
  data: theta1 input; theta2 input; r output; phi output
function [r,phi] = Position(theta1,theta2)
%POSITION
%    [R,PHI] = POSITION(THETA1,THETA2)

%    This function was generated by the Symbolic Math Toolbox version 8.6.
%    17-May-2022 09:32:07

r = sqrt((cos(acos(sqrt((sin(theta1-pi./2.0).*(7.0./4.0e+1)+sin(theta2+pi./2.0).*(7.0./4.0e+1)).^2+abs(cos(theta1-pi./2.0).*(7.0./4.0e+1)+cos(theta2+pi./2.0).*(7.0./4.0e+1)+3.0./2.5e+1).^2).*(5.0./3.0))+atan2(sin(theta1-pi./2.0).*(-7.0./4.0e+1)-sin(theta2+pi./2.0).*(7.0./4.0e+1),abs(cos(theta1-pi./2.0).*(7.0./4.0e+1)+cos(theta2+pi./2.0).*(7.0./4.0e+1)+3.0./2.5e+1))+6.012387278395987e-2).*(-3.328470665197855e-1)+cos(theta2+pi./2.0).*(7.0./4.0e+1)+3.0./5.0e+1).^2+(sin(acos(sqrt((sin(theta1-pi./2.0).*(7.0./4.0e+1)+sin(theta2+pi./2.0).*(7.0./4.0e+1)).^2+abs(cos(theta1-pi./2.0).*(7.0./4.0e+1)+cos(theta2+pi./2.0).*(7.0./4.0e+1)+3.0./2.5e+1).^2).*(5.0./3.0))+atan2(sin(theta1-pi./2.0).*(-7.0./4.0e+1)-sin(theta2+pi./2.0).*(7.0./4.0e+1),abs(cos(theta1-pi./2.0).*(7.0./4.0e+1)+cos(theta2+pi./2.0).*(7.0./4.0e+1)+3.0./2.5e+1))+6.012387278395987e-2).*3.328470665197855e-1+sin(theta2+pi./2.0).*(7.0./4.0e+1)).^2);
if nargout > 1
    phi = pi./2.0-angle(cos(acos(sqrt((sin(theta1-pi./2.0).*(7.0./4.0e+1)+sin(theta2+pi./2.0).*(7.0./4.0e+1)).^2+abs(cos(theta1-pi./2.0).*(7.0./4.0e+1)+cos(theta2+pi./2.0).*(7.0./4.0e+1)+3.0./2.5e+1).^2).*(5.0./3.0))+atan2(sin(theta1-pi./2.0).*(-7.0./4.0e+1)-sin(theta2+pi./2.0).*(7.0./4.0e+1),abs(cos(theta1-pi./2.0).*(7.0./4.0e+1)+cos(theta2+pi./2.0).*(7.0./4.0e+1)+3.0./2.5e+1))+6.012387278395987e-2).*(-3.328470665197855e-1)+sin(acos(sqrt((sin(theta1-pi./2.0).*(7.0./4.0e+1)+sin(theta2+pi./2.0).*(7.0./4.0e+1)).^2+abs(cos(theta1-pi./2.0).*(7.0./4.0e+1)+cos(theta2+pi./2.0).*(7.0./4.0e+1)+3.0./2.5e+1).^2).*(5.0./3.0))+atan2(sin(theta1-pi./2.0).*(-7.0./4.0e+1)-sin(theta2+pi./2.0).*(7.0./4.0e+1),abs(cos(theta1-pi./2.0).*(7.0./4.0e+1)+cos(theta2+pi./2.0).*(7.0./4.0e+1)+3.0./2.5e+1))+6.012387278395987e-2).*3.328470665197855e-1i+cos(theta2+pi./2.0).*(7.0./4.0e+1)+sin(theta2+pi./2.0).*1.75e-1i+3.0./5.0e+1);
end

== matlab function test/MATLAB Function2 ==
  data: w output; E input; dE input
function w  = Controller(E,dE)
    Kp_r = 500;  
    Kp_phi = 20;  
    Kd_r = 10;  
    Kd_phi = 0.1;

    wr = Kp_r*E(1) + Kd_r*dE(1);
    wphi = Kp_phi*E(2) + Kd_phi*dE(2);
    
    w = [wr;wphi];
end

== matlab function test/MATLAB Function4 ==
  data: r_check input; tau1_new output; tau2_new output; w input; JT11 input; JT12 input; JT21 input; JT22 input
function [tau1_new,tau2_new]  = Mapping(r_check,w,JT11,JT12,JT21,JT22)
    JT = [JT11,JT12;JT21,JT22];
    Fpush = 50;
    % foot force - if r is below some value add 100N (at least 62N)
    if r_check<0.36
        tau1_new = JT11*(w(1)+Fpush) + JT12*w(2);
        tau2_new = JT21*(w(1)+Fpush) + JT22*w(2);
    else
        tau1_new = JT11*w(1) + JT12*w(2);
        tau2_new = JT21*w(1) + JT22*w(2);
    end
%        
%     Fext = 20;
%     tau1 = JT11*w(1) + JT12*w(2);
%     tau2 = JT21*w(1) + JT22*w(2);
%     
%     tau = JT*w;
%     tau1_o = tau(1);
%     tau2_o = tau(2);
end
